simulink model "Trafficlightsys"  (R2020a)
settings: Solver=VariableStepAuto  StartTime=0.0  StopTime=10.0  RelTol=1e-3
libraries: simulink x1
settings Model: Creator=USER  LastModifiedBy=USER

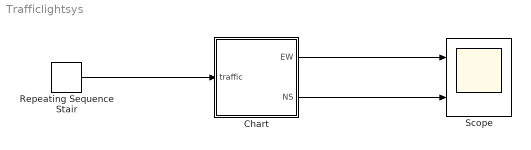
== system Trafficlightsys ==
  Chart : Stateflow chart  TreatAsAtomicUnit=on
  Repeating Sequence Stair : simulink/Sources/Repeating Sequence Stair  OutValues=[3 1 4 2 1].'  tsamp=-1  OutMin=[]  OutMax=[]  OutDataTypeStr=double  OutputDataTypeScalingMode=double  OutDataType=fixdt(0,8)  ConRadixGroup=Best Precision: Vector-wise  OutScaling=2^-12
  Scope : Scope  NumInputPorts=2
  wires:
  Chart/1(EW) -> Scope/1
  Chart/2(NS) -> Scope/2
  Repeating Sequence Stair/1 -> Chart/1(traffic)

== stateflow chart Trafficlightsys/Chart ==
  settings: stateMachineType=MOORE_MACHINE
  state Stop
    EW=red;
    NS=green;
  state NotrafficEW
    EW=red;
    NS=green;
  state PreparetoGo
    EW=red;
    NS=yellow;
  state Go
    EW=green;
    NS=red;
  state PreparetoStop
    EW=yellow;
    NS=red;
  (default) -> Stop
  Stop -> NotrafficEW : after(20,tick)
  NotrafficEW -> PreparetoGo : [traffic==1]
  PreparetoGo -> Go : after(5,tick)
  PreparetoStop -> Stop : after(5,tick)
  Go -> PreparetoStop : after(10,tick)
  data: EW output; NS output; red constant double =1; yellow constant double =2; traffic input double; green constant double =3
